simulink model "Edge_trig_counter"  (R2020a)
settings: Solver=VariableStepAuto  StartTime=0.0  StopTime=10.0  RelTol=1e-3
settings Model: Creator=anony  LastModifiedBy=anony

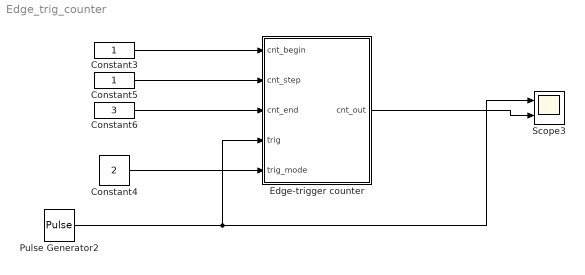
== system Edge_trig_counter ==
  Constant3 : Constant
  Constant4 : Constant  Value=2
  Constant5 : Constant
  Constant6 : Constant  Value=3
  Edge-trigger counter : MATLAB Function  TreatAsAtomicUnit=on  SystemSampleTime=50e-6
  Pulse Generator2 : DiscretePulseGenerator  PulseType=Time based  Period=1  PulseWidth=10
  Scope3 : Scope  NumInputPorts=2
  wires:
  Edge-trigger counter/1(cnt_out) -> Scope3/2
  Constant6/1 -> Edge-trigger counter/3(cnt_end)
  Constant5/1 -> Edge-trigger counter/2(cnt_step)
  Constant3/1 -> Edge-trigger counter/1(cnt_begin)
  Constant4/1 -> Edge-trigger counter/5(trig_mode)
  Pulse Generator2/1 -> Scope3/1, Edge-trigger counter/4(trig)

== matlab function Edge_trig_counter/Edge-trigger counter ==
  data: cnt_begin input; cnt_step input; cnt_end input; trig input; trig_mode input; cnt_out output
function cnt_out = fcn(cnt_begin, cnt_step, cnt_end, trig, trig_mode)
% trig_mode: 1 for rising-edge trigger, 2 for falling-edge trigger;
% static var declaration
persistent trig_now trig_last  rise_trig fall_trig cnt
    if isempty(trig_now)
        trig_now = 0;
    end

    if isempty(trig_last)
        trig_last = 0;
    end
    
    if isempty(rise_trig)
        rise_trig = 0;
    end
    
    if isempty(fall_trig)
        fall_trig = 0;
    end
    
    if isempty(trig_mode)
        trig_mode = 0;
    end
    
    if isempty(cnt)
        cnt = cnt_begin;
    end

% Event catch depend on trig_mode
trig_now = trig;
if trig_now ~= trig_last
    if trig_now > trig_last
        if trig_mode == 1
            rise_trig = 1;
            % Your code here...
        end
    elseif trig_now < trig_last
        if trig_mode == 2
            fall_trig = 1;
            % Your code here...
            cnt = cnt + cnt_step;
            if cnt > cnt_end
                cnt = cnt_begin;
            end
        end
    end
end

trig_last = trig_now;

cnt_out = cnt
